simulink model "Problem_"  (R2020b)
settings: Solver=VariableStepAuto  StartTime=0.0  StopTime=10.0  RelTol=1e-3
values from neighbouring files (symbols this model uses):
  L = 0.335    [p.m]
settings Model: Creator=HP  LastModifiedBy=HP

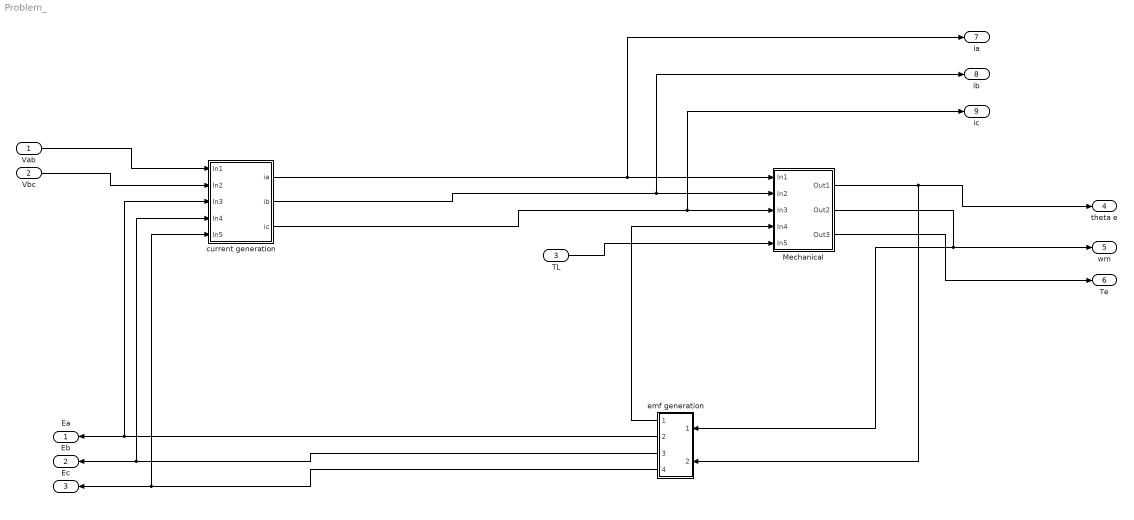
== system Problem_ ==
  Vab : Inport
  Vbc : Inport  Port=2
  TL : Inport  Port=3
  Mechanical : Subsystem
  current generation : Subsystem
  emf generation : Subsystem
  Ea : Outport
  Eb : Outport  Port=2
  Ec : Outport  Port=3
  theta e : Outport  Port=4
  wm : Outport  Port=5
  Te : Outport  Port=6
  ia : Outport  Port=7
  ib : Outport  Port=8
  ic : Outport  Port=9
  wires:
  current generation/1(ia) -> ia/1, Mechanical/1(In1)
  emf generation/3(Out3) -> current generation/4(In4), Eb/1
  TL/1 -> Mechanical/5(In5)
  emf generation/4(Out4) -> current generation/5(In5), Ec/1
  current generation/2(ib) -> ib/1, Mechanical/2(In2)
  Mechanical/1(Out1) -> emf generation/2(In2), theta e/1
  current generation/3(ic) -> Mechanical/3(In3), ic/1
  Mechanical/3(Out3) -> Te/1
  emf generation/1(Out1) -> Mechanical/4(In4)
  emf generation/2(Out2) -> current generation/3(In3), Ea/1
  Vab/1 -> current generation/1(In1)
  Vbc/1 -> current generation/2(In2)
  Mechanical/2(Out2) -> wm/1, emf generation/1(In1)

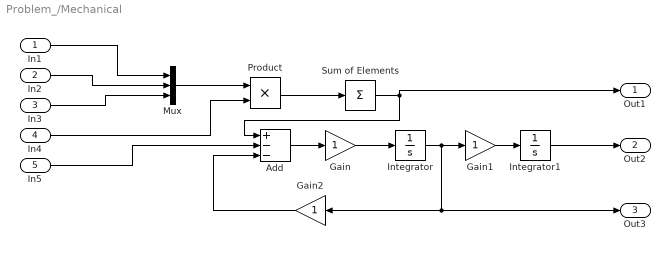
== system Problem_/Mechanical ==
  In1 : Inport
  In2 : Inport  Port=2
  In3 : Inport  Port=3
  In4 : Inport  Port=4
  In5 : Inport  Port=5
  Add : Sum  Inputs=+--
  Gain : Gain
  Gain1 : Gain
  Gain2 : Gain
  Integrator : Integrator
  Integrator1 : Integrator
  Mux : Mux  Inputs=3
  Product : Product
  Sum of Elements : Sum  Inputs=+
  Out1 : Outport
  Out2 : Outport  Port=2
  Out3 : Outport  Port=3
  wires:
  Integrator/1 -> Out3/1, Gain2/1, Gain1/1
  Add/1 -> Gain/1
  Gain/1 -> Integrator/1
  Mux/1 -> Product/1
  Gain1/1 -> Integrator1/1
  In1/1 -> Mux/1
  Product/1 -> Sum of Elements/1
  Sum of Elements/1 -> Out1/1, Add/1
  In2/1 -> Mux/2
  In5/1 -> Add/2
  Gain2/1 -> Add/3
  In4/1 -> Product/2
  Integrator1/1 -> Out2/1
  In3/1 -> Mux/3

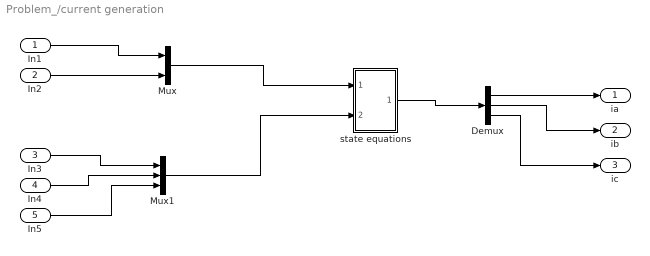
== system Problem_/current generation ==
  In1 : Inport
  In2 : Inport  Port=2
  In3 : Inport  Port=3
  In4 : Inport  Port=4
  In5 : Inport  Port=5
  Demux : Demux  Outputs=3
  Mux : Mux  Inputs=2
  Mux1 : Mux  Inputs=3
  state equations : Subsystem
  ia : Outport
  ib : Outport  Port=2
  ic : Outport  Port=3
  wires:
  Mux1/1 -> state equations/2(In2)
  Mux/1 -> state equations/1(In1)
  In4/1 -> Mux1/2
  In2/1 -> Mux/2
  In1/1 -> Mux/1
  In3/1 -> Mux1/1
  state equations/1(Out1) -> Demux/1
  Demux/3 -> ic/1
  Demux/2 -> ib/1
  Demux/1 -> ia/1
  In5/1 -> Mux1/3

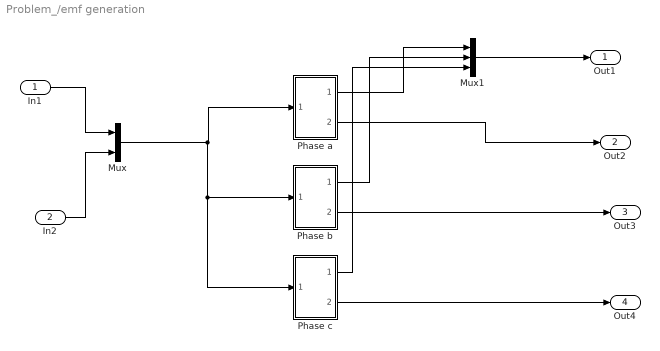
== system Problem_/emf generation ==
  In1 : Inport
  In2 : Inport  Port=2
  Mux : Mux  Inputs=2
  Mux1 : Mux  Inputs=3
  Phase a : Subsystem
  Phase b : Subsystem
  Phase c : Subsystem
  Out1 : Outport
  Out2 : Outport  Port=2
  Out3 : Outport  Port=3
  Out4 : Outport  Port=4
  wires:
  In2/1 -> Mux/2
  In1/1 -> Mux/1
  Mux/1 -> Phase c/1(In1), Phase b/1(In1), Phase a/1(In1)
  Phase c/2(Out2) -> Out4/1
  Mux1/1 -> Out1/1
  Phase a/1(Out1) -> Mux1/1
  Phase c/1(Out1) -> Mux1/3
  Phase b/1(Out1) -> Mux1/2
  Phase b/2(Out2) -> Out3/1
  Phase a/2(Out2) -> Out2/1

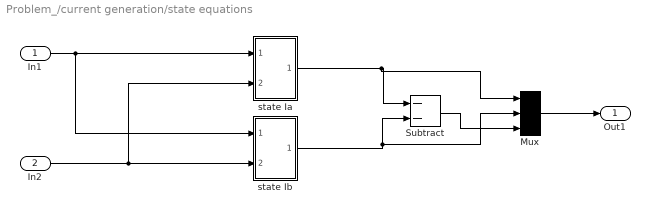
== system Problem_/current generation/state equations ==
  In1 : Inport
  In2 : Inport  Port=2
  Mux : Mux  Inputs=3
  Subtract : Sum  Inputs=--
  state Ia : Subsystem
  state Ib : Subsystem
  Out1 : Outport
  wires:
  In1/1 -> state Ib/1(Vab,Vbc), state Ia/1(In1)
  Mux/1 -> Out1/1
  In2/1 -> state Ib/2(Eabc), state Ia/2(In2)
  Subtract/1 -> Mux/3
  state Ib/1(Out1) -> Mux/2, Subtract/2
  state Ia/1(Out1) -> Mux/1, Subtract/1

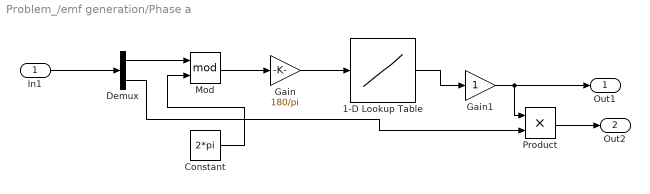
== system Problem_/emf generation/Phase a ==
  In1 : Inport
  1-D Lookup Table : Lookup_n-D  NumberOfTableDimensions=1  BreakpointsForDimension1=[-5:5]  Table=tanh([-5:5])  InternalRulePriority=Speed  RndMeth=Simplest  InputSameDT=on
  Constant : Constant  Value=2*pi
  Demux : Demux  Outputs=2
  Gain : Gain  Gain=180/pi
  Gain1 : Gain
  Mod : Math  Operator=mod  SaturateOnIntegerOverflow=on
  Product : Product
  Out1 : Outport
  Out2 : Outport  Port=2
  wires:
  Product/1 -> Out2/1
  1-D Lookup Table/1 -> Gain1/1
  In1/1 -> Demux/1
  Demux/2 -> Product/2
  Demux/1 -> Mod/1
  Gain1/1 -> Out1/1, Product/1
  Gain/1 -> 1-D Lookup Table/1
  Constant/1 -> Mod/2
  Mod/1 -> Gain/1

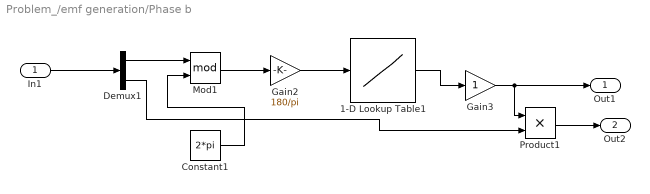
== system Problem_/emf generation/Phase b ==
  In1 : Inport
  1-D Lookup Table1 : Lookup_n-D  NumberOfTableDimensions=1  BreakpointsForDimension1=[-5:5]  Table=tanh([-5:5])  InternalRulePriority=Speed  RndMeth=Simplest  InputSameDT=on
  Constant1 : Constant  Value=2*pi
  Demux1 : Demux  Outputs=2
  Gain2 : Gain  Gain=180/pi
  Gain3 : Gain
  Mod1 : Math  Operator=mod  SaturateOnIntegerOverflow=on
  Product1 : Product
  Out1 : Outport
  Out2 : Outport  Port=2
  wires:
  Gain2/1 -> 1-D Lookup Table1/1
  Demux1/2 -> Product1/2
  Constant1/1 -> Mod1/2
  Gain3/1 -> Out1/1, Product1/1
  Mod1/1 -> Gain2/1
  1-D Lookup Table1/1 -> Gain3/1
  Demux1/1 -> Mod1/1
  Product1/1 -> Out2/1
  In1/1 -> Demux1/1

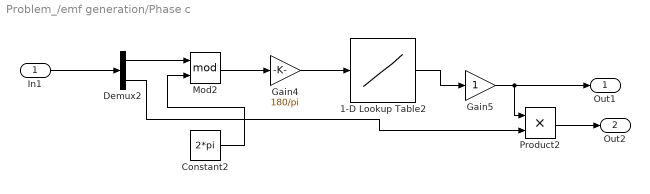
== system Problem_/emf generation/Phase c ==
  In1 : Inport
  1-D Lookup Table2 : Lookup_n-D  NumberOfTableDimensions=1  BreakpointsForDimension1=[-5:5]  Table=tanh([-5:5])  InternalRulePriority=Speed  RndMeth=Simplest  InputSameDT=on
  Constant2 : Constant  Value=2*pi
  Demux2 : Demux  Outputs=2
  Gain4 : Gain  Gain=180/pi
  Gain5 : Gain
  Mod2 : Math  Operator=mod  SaturateOnIntegerOverflow=on
  Product2 : Product
  Out1 : Outport
  Out2 : Outport  Port=2
  wires:
  Gain5/1 -> Out1/1, Product2/1
  Demux2/1 -> Mod2/1
  Mod2/1 -> Gain4/1
  1-D Lookup Table2/1 -> Gain5/1
  In1/1 -> Demux2/1
  Gain4/1 -> 1-D Lookup Table2/1
  Demux2/2 -> Product2/2
  Constant2/1 -> Mod2/2
  Product2/1 -> Out2/1

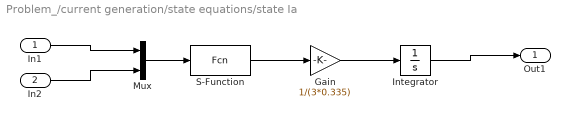
== system Problem_/current generation/state equations/state Ia ==
  In1 : Inport
  In2 : Inport  Port=2
  Gain : Gain  Gain=1/(3*0.335)
  Integrator : Integrator
  Mux : Mux  Inputs=2
  S-Function : S-Function  FunctionName=Fcn  SFunctionDeploymentMode=off  EnableBusSupport=off
  Out1 : Outport
  wires:
  S-Function/1 -> Gain/1
  In2/1 -> Mux/2
  Mux/1 -> S-Function/1
  Gain/1 -> Integrator/1
  In1/1 -> Mux/1
  Integrator/1 -> Out1/1

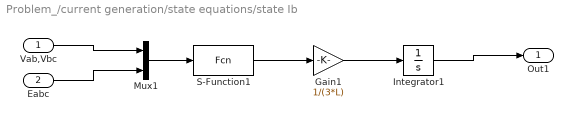
== system Problem_/current generation/state equations/state Ib ==
  Vab,Vbc : Inport
  Eabc : Inport  Port=2
  Gain1 : Gain  Gain=1/(3*L)
  Integrator1 : Integrator
  Mux1 : Mux  Inputs=2
  S-Function1 : S-Function  FunctionName=Fcn  SFunctionDeploymentMode=off  EnableBusSupport=off
  Out1 : Outport
  wires:
  Eabc/1 -> Mux1/2
  Mux1/1 -> S-Function1/1
  Gain1/1 -> Integrator1/1
  S-Function1/1 -> Gain1/1
  Integrator1/1 -> Out1/1
  Vab,Vbc/1 -> Mux1/1
